simulink subsystem "Sim_Plots"  (R2024b)
settings: Solver=VariableStepAuto  StartTime=0.0  StopTime=10.0  RelTol=1e-3
undefined symbols (not defined in the file or in its folder): SimIn
settings Model: Creator=bmsimmon  LastModifiedBy=macheson
settings RTWCC: GPUComputeCapability=3.5

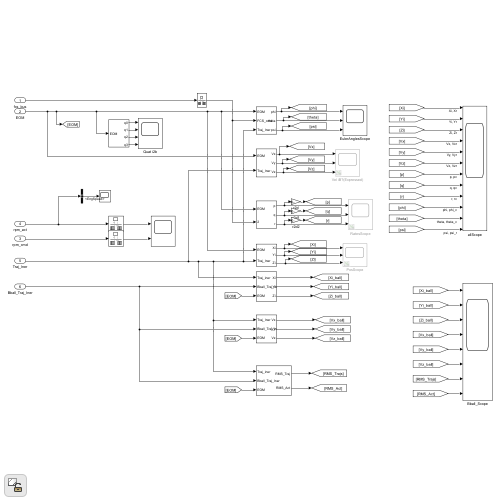
[thumbnail: Simulink's stored preview of the top-level diagram]
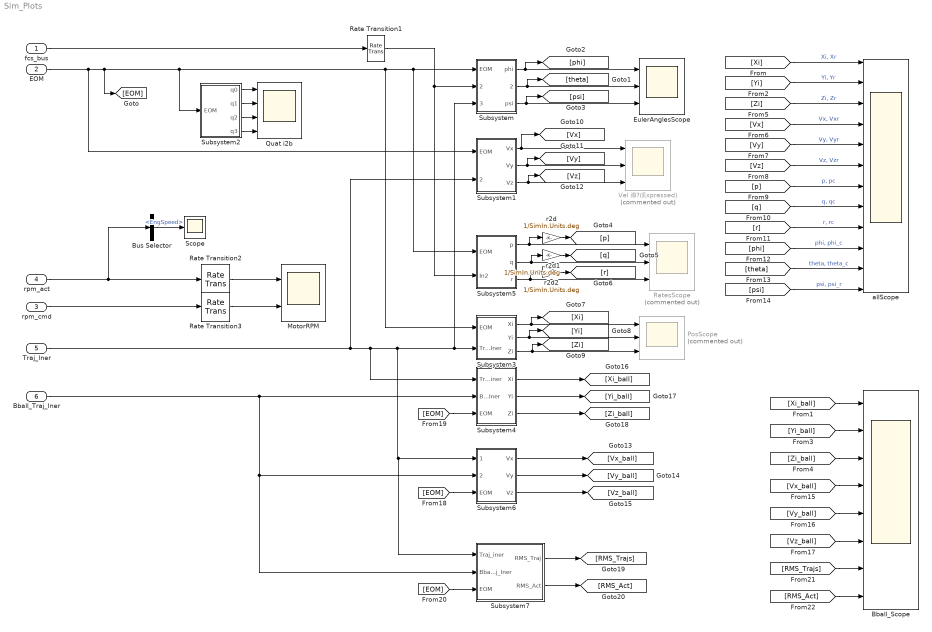
== system Sim_Plots ==
  fcs_bus : Inport
  EOM : Inport  Port=2
  rpm_cmd : Inport  Port=3
  rpm_act : Inport  Port=4
  Traj_Iner : Inport  Port=5
  Bball_Traj_Iner : Inport  Port=6
  Bball_Scope : Scope  NumInputPorts=8
  Bus Selector : BusSelector  OutputSignals=EngSpeed
  EulerAnglesScope : Scope  NumInputPorts=3
  MotorRPM : Scope  NumInputPorts=2
  PosScope : Scope  Commented=on  NumInputPorts=3
  Quat i2b : Scope  NumInputPorts=4
  Rate Transition1 : RateTransition
  Rate Transition2 : RateTransition
  Rate Transition3 : RateTransition
  RatesScope : Scope  Commented=on  NumInputPorts=3
  Scope : Scope
  Subsystem : Subsystem
  Subsystem1 : Subsystem
  Subsystem2 : Subsystem
  Subsystem3 : Subsystem
  Subsystem4 : Subsystem
  Subsystem5 : Subsystem
  Subsystem6 : Subsystem
  Subsystem7 : Subsystem
  Vel iB?(Expressed) : Scope  Commented=on  NumInputPorts=3
  allScope : Scope  NumInputPorts=12
  r2d : Gain  Gain=1/SimIn.Units.deg
  r2d1 : Gain  Gain=1/SimIn.Units.deg
  r2d2 : Gain  Gain=1/SimIn.Units.deg
  wires:
  Subsystem/1(phi) -> EulerAnglesScope/1, [phi]
  Subsystem/2(theta) -> EulerAnglesScope/2, [theta]
  Subsystem/3(psi) -> EulerAnglesScope/3, [psi]
  Subsystem2/1(q0) -> Quat i2b/1
  Subsystem2/2(q1) -> Quat i2b/2
  Subsystem2/3(q2) -> Quat i2b/3
  Subsystem2/4(q3) -> Quat i2b/4
  Subsystem1/1(Vx) -> Vel iB?(Expressed)/1, [Vx]
  Subsystem1/2(Vy) -> Vel iB?(Expressed)/2, [Vy]
  Subsystem1/3(Vz) -> Vel iB?(Expressed)/3, [Vz]
  Subsystem3/2(Yi) -> PosScope/2, [Yi]
  Subsystem3/3(Zi) -> PosScope/3, [Zi]
  Subsystem3/1(Xi) -> PosScope/1, [Xi]
  Subsystem5/1(p) -> RatesScope/1, r2d/1
  Subsystem5/2(q) -> RatesScope/2, r2d1/1
  Subsystem5/3(r) -> RatesScope/3, r2d2/1
  rpm_cmd/1 -> Rate Transition3/1
  rpm_act/1 -> Rate Transition2/1, Bus Selector/1
  Rate Transition2/1 -> MotorRPM/1
  [Xi] -> allScope/1  "Xi, Xr"
  [Yi] -> allScope/2  "Yi, Yr"
  [Zi] -> allScope/3  "Zi, Zr"
  [Vx] -> allScope/4  "Vx, Vxr"
  [Vy] -> allScope/5  "Vy, Vyr"
  [Vz] -> allScope/6  "Vz, Vzr"
  [p] -> allScope/7  "p, pc"
  [q] -> allScope/8  "q, qc"
  [r] -> allScope/9  "r, rc"
  [phi] -> allScope/10  "phi, phi_c"
  [theta] -> allScope/11  "theta, theta_c"
  [psi] -> allScope/12  "psi, psi_r"
  r2d/1 -> [p]
  r2d1/1 -> [q]
  r2d2/1 -> [r]
  Rate Transition1/1 -> Subsystem5/2(In2), Subsystem/2(FCS_cmd)
  fcs_bus/1 -> Rate Transition1/1
  Rate Transition3/1 -> MotorRPM/2
  EOM/1 -> Subsystem/1(EOM), Subsystem5/1(EOM), Subsystem3/1(EOM), Subsystem2/1(EOM), [EOM], Subsystem1/1(EOM)
  Bus Selector/1 -> Scope/1  "<EngSpeed>"
  Subsystem6/1(Vx) -> [Vx_ball]
  Subsystem6/2(Vy) -> [Vy_ball]
  Subsystem6/3(Vz) -> [Vz_ball]
  Subsystem4/1(Xi) -> [Xi_ball]
  Subsystem4/2(Yi) -> [Yi_ball]
  Subsystem4/3(Zi) -> [Zi_ball]
  [Xi_ball] -> Bball_Scope/1
  [Yi_ball] -> Bball_Scope/2
  [Zi_ball] -> Bball_Scope/3
  [Vx_ball] -> Bball_Scope/4
  [Vy_ball] -> Bball_Scope/5
  [Vz_ball] -> Bball_Scope/6
  [EOM] -> Subsystem6/3(EOM)
  [EOM] -> Subsystem4/3(EOM)
  Bball_Traj_Iner/1 -> Subsystem4/2(Bball_Traj_Iner), Subsystem6/2(Bball_Traj_Iner), Subsystem7/2(Bball_Traj_Iner)
  [EOM] -> Subsystem7/3(EOM)
  Traj_Iner/1 -> Subsystem3/2(Traj_Iner), Subsystem/3(Traj_Iner), Subsystem6/1(Traj_Iner), Subsystem7/1(Traj_iner), Subsystem4/1(Traj_iner), Subsystem1/2(Traj_Iner)
  Subsystem7/1(RMS_Traj) -> [RMS_Trajs]
  Subsystem7/2(RMS_Act) -> [RMS_Act]
  [RMS_Trajs] -> Bball_Scope/7
  [RMS_Act] -> Bball_Scope/8

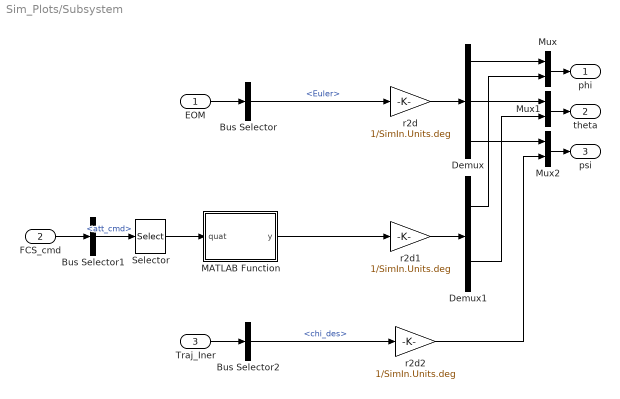
== system Sim_Plots/Subsystem ==
  EOM : Inport
  FCS_cmd : Inport  Port=2
  Traj_Iner : Inport  Port=3
  Bus Selector : BusSelector  OutputSignals=WorldRelativeData.Euler
  Bus Selector1 : BusSelector  OutputSignals=fcs_data.fcs_data_baseline.IL_fcs_data.att_cmd
  Bus Selector2 : BusSelector  OutputSignals=chi_des
  Demux : Demux  Outputs=3
  Demux1 : Demux  Outputs=2
  MATLAB Function : MATLAB Function  TreatAsAtomicUnit=on
  Mux : Mux  Inputs=2
  Mux1 : Mux  Inputs=2
  Mux2 : Mux  Inputs=2
  Selector : Selector  InputPortWidth=5  IndexOptions=Index vector (dialog)  Indices=[1:4]  OutputSizes=1
  r2d : Gain  Gain=1/SimIn.Units.deg
  r2d1 : Gain  Gain=1/SimIn.Units.deg
  r2d2 : Gain  Gain=1/SimIn.Units.deg
  phi : Outport  VectorParamsAs1DForOutWhenUnconnected=off
  theta : Outport  Port=2  VectorParamsAs1DForOutWhenUnconnected=off
  psi : Outport  Port=3  VectorParamsAs1DForOutWhenUnconnected=off
  wires:
  MATLAB Function/1(y) -> r2d1/1
  r2d2/1 -> Mux2/2
  Bus Selector2/1 -> r2d2/1  "<chi_des>"
  Mux2/1 -> psi/1
  Traj_Iner/1 -> Bus Selector2/1
  r2d1/1 -> Demux1/1
  Bus Selector1/1 -> Selector/1  "<att_cmd>"
  Selector/1 -> MATLAB Function/1(quat)
  Demux/3 -> Mux2/1
  Demux1/2 -> Mux1/2
  Mux1/1 -> theta/1
  Demux/2 -> Mux1/1
  Demux1/1 -> Mux/2
  Mux/1 -> phi/1
  FCS_cmd/1 -> Bus Selector1/1
  Demux/1 -> Mux/1
  r2d/1 -> Demux/1
  EOM/1 -> Bus Selector/1
  Bus Selector/1 -> r2d/1  "<Euler>"

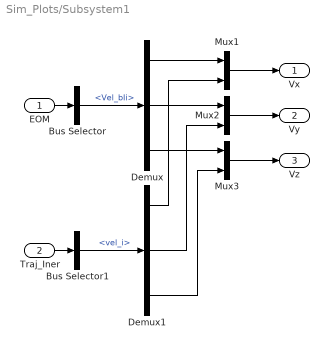
== system Sim_Plots/Subsystem1 ==
  EOM : Inport
  Traj_Iner : Inport  Port=2
  Bus Selector : BusSelector  OutputSignals=InertialData.Vel_bIi
  Bus Selector1 : BusSelector  OutputSignals=vel_i
  Demux : Demux  Outputs=3
  Demux1 : Demux  Outputs=3
  Mux1 : Mux  Inputs=2
  Mux2 : Mux  Inputs=2
  Mux3 : Mux  Inputs=2
  Vx : Outport  VectorParamsAs1DForOutWhenUnconnected=off
  Vy : Outport  Port=2  VectorParamsAs1DForOutWhenUnconnected=off
  Vz : Outport  Port=3  VectorParamsAs1DForOutWhenUnconnected=off
  wires:
  Demux1/3 -> Mux3/2
  Demux1/2 -> Mux2/2
  Demux1/1 -> Mux1/2
  Bus Selector1/1 -> Demux1/1  "<vel_i>"
  Traj_Iner/1 -> Bus Selector1/1
  Mux3/1 -> Vz/1
  Mux2/1 -> Vy/1
  Mux1/1 -> Vx/1
  Demux/2 -> Mux2/1
  Bus Selector/1 -> Demux/1  "<Vel_bIi>"
  Demux/3 -> Mux3/1
  Demux/1 -> Mux1/1
  EOM/1 -> Bus Selector/1

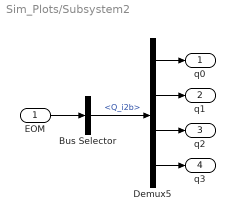
== system Sim_Plots/Subsystem2 ==
  EOM : Inport
  Bus Selector : BusSelector  OutputSignals=InertialData.Q_i2b
  Demux5 : Demux
  q0 : Outport  VectorParamsAs1DForOutWhenUnconnected=off
  q1 : Outport  Port=2  VectorParamsAs1DForOutWhenUnconnected=off
  q2 : Outport  Port=3  VectorParamsAs1DForOutWhenUnconnected=off
  q3 : Outport  Port=4  VectorParamsAs1DForOutWhenUnconnected=off
  wires:
  Demux5/4 -> q3/1
  Demux5/3 -> q2/1
  Demux5/2 -> q1/1
  Demux5/1 -> q0/1
  EOM/1 -> Bus Selector/1
  Bus Selector/1 -> Demux5/1  "<Q_i2b>"

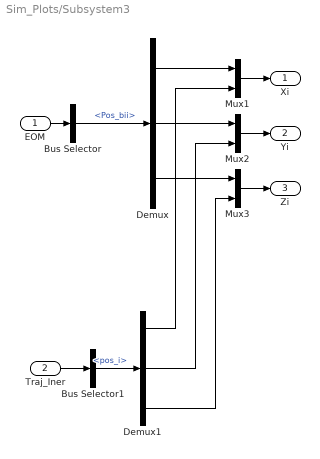
== system Sim_Plots/Subsystem3 ==
  EOM : Inport
  Traj_Iner : Inport  Port=2
  Bus Selector : BusSelector  OutputSignals=InertialData.Pos_bii
  Bus Selector1 : BusSelector  OutputSignals=pos_i
  Demux : Demux  Outputs=3
  Demux1 : Demux  Outputs=3
  Mux1 : Mux  Inputs=2
  Mux2 : Mux  Inputs=2
  Mux3 : Mux  Inputs=2
  Xi : Outport  VectorParamsAs1DForOutWhenUnconnected=off
  Yi : Outport  Port=2  VectorParamsAs1DForOutWhenUnconnected=off
  Zi : Outport  Port=3  VectorParamsAs1DForOutWhenUnconnected=off
  wires:
  Demux1/3 -> Mux3/2
  Mux3/1 -> Zi/1
  Demux1/2 -> Mux2/2
  Mux2/1 -> Yi/1
  Demux1/1 -> Mux1/2
  Mux1/1 -> Xi/1
  Bus Selector1/1 -> Demux1/1  "<pos_i>"
  Traj_Iner/1 -> Bus Selector1/1
  Demux/2 -> Mux2/1
  Demux/3 -> Mux3/1
  Demux/1 -> Mux1/1
  EOM/1 -> Bus Selector/1
  Bus Selector/1 -> Demux/1  "<Pos_bii>"

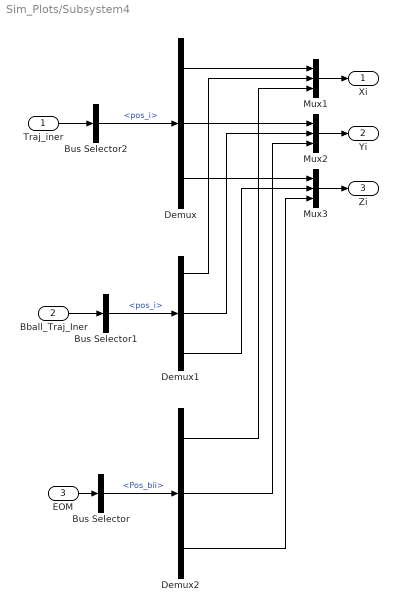
== system Sim_Plots/Subsystem4 ==
  Traj_iner : Inport
  Bball_Traj_Iner : Inport  Port=2
  EOM : Inport  Port=3
  Bus Selector : BusSelector  OutputSignals=InertialData.Pos_bii
  Bus Selector1 : BusSelector  OutputSignals=pos_i
  Bus Selector2 : BusSelector  OutputSignals=pos_i
  Demux : Demux  Outputs=3
  Demux1 : Demux  Outputs=3
  Demux2 : Demux  Outputs=3
  Mux1 : Mux  Inputs=3
  Mux2 : Mux  Inputs=3
  Mux3 : Mux  Inputs=3
  Xi : Outport  VectorParamsAs1DForOutWhenUnconnected=off
  Yi : Outport  Port=2  VectorParamsAs1DForOutWhenUnconnected=off
  Zi : Outport  Port=3  VectorParamsAs1DForOutWhenUnconnected=off
  wires:
  Bus Selector/1 -> Demux2/1  "<Pos_bii>"
  Demux2/1 -> Mux1/3
  Demux2/3 -> Mux3/3
  Demux2/2 -> Mux2/3
  EOM/1 -> Bus Selector/1
  Demux1/3 -> Mux3/2
  Mux3/1 -> Zi/1
  Demux1/2 -> Mux2/2
  Mux2/1 -> Yi/1
  Demux1/1 -> Mux1/2
  Mux1/1 -> Xi/1
  Bus Selector1/1 -> Demux1/1  "<pos_i>"
  Bball_Traj_Iner/1 -> Bus Selector1/1
  Demux/2 -> Mux2/1
  Demux/3 -> Mux3/1
  Demux/1 -> Mux1/1
  Traj_iner/1 -> Bus Selector2/1
  Bus Selector2/1 -> Demux/1  "<pos_i>"

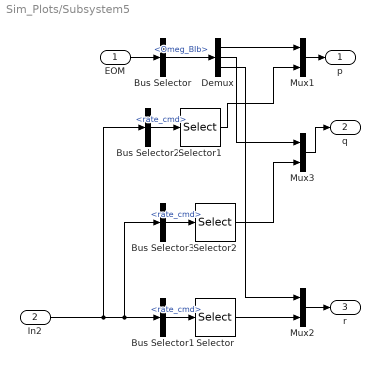
== system Sim_Plots/Subsystem5 ==
  EOM : Inport
  In2 : Inport  Port=2
  Bus Selector : BusSelector  OutputSignals=InertialData.Omeg_BIb
  Bus Selector1 : BusSelector  OutputSignals=fcs_data.fcs_data_baseline.IL_fcs_data.rate_cmd
  Bus Selector2 : BusSelector  OutputSignals=fcs_data.fcs_data_baseline.IL_fcs_data.rate_cmd
  Bus Selector3 : BusSelector  OutputSignals=fcs_data.fcs_data_baseline.IL_fcs_data.rate_cmd
  Demux : Demux  Outputs=3
  Mux1 : Mux  Inputs=2
  Mux2 : Mux  Inputs=2
  Mux3 : Mux  Inputs=2
  Selector : Selector  InputPortWidth=4  IndexOptions=Index vector (dialog)  Indices=[3]  OutputSizes=1
  Selector1 : Selector  InputPortWidth=4  IndexOptions=Index vector (dialog)  Indices=1  OutputSizes=1
  Selector2 : Selector  InputPortWidth=4  IndexOptions=Index vector (dialog)  Indices=2  OutputSizes=1
  p : Outport  VectorParamsAs1DForOutWhenUnconnected=off
  q : Outport  Port=2  VectorParamsAs1DForOutWhenUnconnected=off
  r : Outport  Port=3  VectorParamsAs1DForOutWhenUnconnected=off
  wires:
  Selector2/1 -> Mux3/2
  Mux3/1 -> q/1
  Bus Selector3/1 -> Selector2/1  "<rate_cmd>"
  In2/1 -> Bus Selector1/1, Bus Selector3/1, Bus Selector2/1
  Selector1/1 -> Mux1/2
  Mux1/1 -> p/1
  Bus Selector2/1 -> Selector1/1  "<rate_cmd>"
  Bus Selector1/1 -> Selector/1  "<rate_cmd>"
  Mux2/1 -> r/1
  Demux/2 -> Mux3/1
  Demux/1 -> Mux1/1
  EOM/1 -> Bus Selector/1
  Selector/1 -> Mux2/2
  Demux/3 -> Mux2/1
  Bus Selector/1 -> Demux/1  "<Omeg_BIb>"

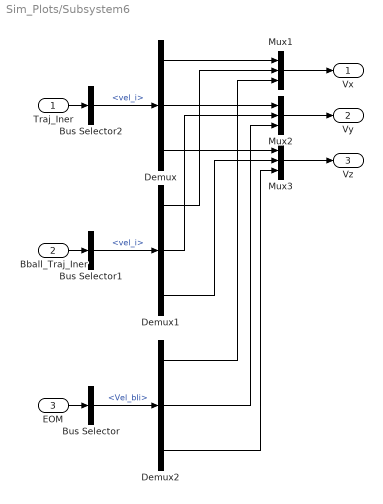
== system Sim_Plots/Subsystem6 ==
  Traj_Iner : Inport
  Bball_Traj_Iner : Inport  Port=2
  EOM : Inport  Port=3
  Bus Selector : BusSelector  OutputSignals=InertialData.Vel_bIi
  Bus Selector1 : BusSelector  OutputSignals=vel_i
  Bus Selector2 : BusSelector  OutputSignals=vel_i
  Demux : Demux  Outputs=3
  Demux1 : Demux  Outputs=3
  Demux2 : Demux  Outputs=3
  Mux1 : Mux  Inputs=3
  Mux2 : Mux  Inputs=3
  Mux3 : Mux  Inputs=3
  Vx : Outport  VectorParamsAs1DForOutWhenUnconnected=off
  Vy : Outport  Port=2  VectorParamsAs1DForOutWhenUnconnected=off
  Vz : Outport  Port=3  VectorParamsAs1DForOutWhenUnconnected=off
  wires:
  Demux2/1 -> Mux1/3
  Demux2/2 -> Mux2/3
  Demux2/3 -> Mux3/3
  Bus Selector/1 -> Demux2/1  "<Vel_bIi>"
  EOM/1 -> Bus Selector/1
  Demux1/3 -> Mux3/2
  Demux1/2 -> Mux2/2
  Demux1/1 -> Mux1/2
  Bus Selector1/1 -> Demux1/1  "<vel_i>"
  Bball_Traj_Iner/1 -> Bus Selector1/1
  Mux3/1 -> Vz/1
  Mux2/1 -> Vy/1
  Mux1/1 -> Vx/1
  Demux/2 -> Mux2/1
  Bus Selector2/1 -> Demux/1  "<vel_i>"
  Demux/3 -> Mux3/1
  Demux/1 -> Mux1/1
  Traj_Iner/1 -> Bus Selector2/1

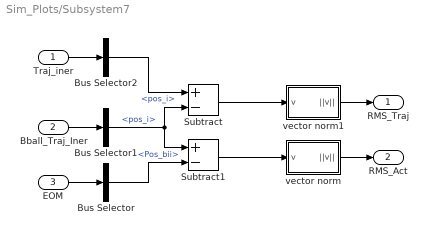
== system Sim_Plots/Subsystem7 ==
  Traj_iner : Inport
  Bball_Traj_Iner : Inport  Port=2
  EOM : Inport  Port=3
  Bus Selector : BusSelector  OutputSignals=InertialData.Pos_bii
  Bus Selector1 : BusSelector  OutputSignals=pos_i
  Bus Selector2 : BusSelector  OutputSignals=pos_i
  Subtract : Sum  Inputs=+-
  Subtract1 : Sum  Inputs=+-
  vector norm : Subsystem
  vector norm1 : Subsystem
  RMS_Traj : Outport  VectorParamsAs1DForOutWhenUnconnected=off
  RMS_Act : Outport  Port=2  VectorParamsAs1DForOutWhenUnconnected=off
  wires:
  Subtract1/1 -> vector norm/1(v)
  Subtract/1 -> vector norm1/1(v)
  vector norm/1(||v||) -> RMS_Act/1
  vector norm1/1(||v||) -> RMS_Traj/1
  Bus Selector2/1 -> Subtract/1  "<pos_i>"
  Bus Selector/1 -> Subtract1/2  "<Pos_bii>"
  EOM/1 -> Bus Selector/1
  Bus Selector1/1 -> Subtract1/1, Subtract/2  "<pos_i>"
  Bball_Traj_Iner/1 -> Bus Selector1/1
  Traj_iner/1 -> Bus Selector2/1

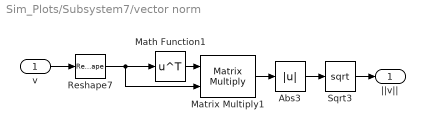
== system Sim_Plots/Subsystem7/vector norm ==
  v : Inport
  Abs3 : Abs  SaturateOnIntegerOverflow=off
  Math Function1 : Math  Operator=transpose  SignedPower=on
  Matrix Multiply1 : Product  Multiplication=Matrix(*)
  Reshape7 : Reshape  OutputDimensionality=Column vector (2-D)
  Sqrt3 : Sqrt
  ||v|| : Outport  VectorParamsAs1DForOutWhenUnconnected=off
  wires:
  Sqrt3/1 -> ||v||/1
  v/1 -> Reshape7/1
  Matrix Multiply1/1 -> Abs3/1
  Math Function1/1 -> Matrix Multiply1/1
  Abs3/1 -> Sqrt3/1
  Reshape7/1 -> Matrix Multiply1/2, Math Function1/1

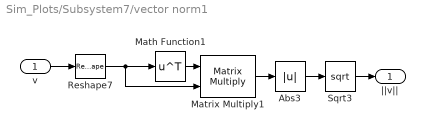
== system Sim_Plots/Subsystem7/vector norm1 ==
  v : Inport
  Abs3 : Abs  SaturateOnIntegerOverflow=off
  Math Function1 : Math  Operator=transpose  SignedPower=on
  Matrix Multiply1 : Product  Multiplication=Matrix(*)
  Reshape7 : Reshape  OutputDimensionality=Column vector (2-D)
  Sqrt3 : Sqrt
  ||v|| : Outport  VectorParamsAs1DForOutWhenUnconnected=off
  wires:
  Sqrt3/1 -> ||v||/1
  v/1 -> Reshape7/1
  Matrix Multiply1/1 -> Abs3/1
  Math Function1/1 -> Matrix Multiply1/1
  Abs3/1 -> Sqrt3/1
  Reshape7/1 -> Matrix Multiply1/2, Math Function1/1

== matlab function Sim_Plots/Subsystem/MATLAB Function ==
  data: quat input; y output
function y = Conv2Euler(quat)

% This function converts from a normalized quat=[w,x,y,z] to Euler angles
% for the body fixed rotation sequence 321

phi = atan2(2*(quat(1)*quat(2)+quat(3)*quat(4)), 1-2*(quat(2)^2+quat(3)^2));
theta = asin(2*(quat(1)*quat(3)-quat(2)*quat(4)));

y = [phi;theta];
